simulink model "MECH6325_HW4_pblm3d"  (R2020a)
settings: Solver=VariableStepAuto  StartTime=0.0  StopTime=10.0  RelTol=1e-3
libraries: simulink x2, cstblocks x1
settings Model: Creator=Jonas  LastModifiedBy=Jonas

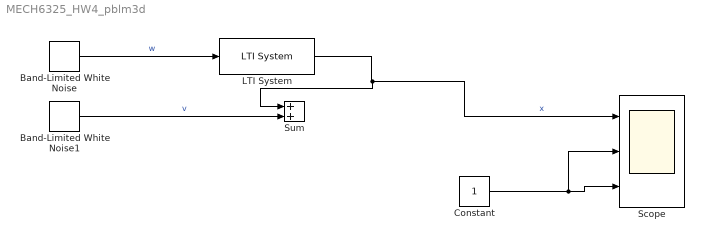
== system MECH6325_HW4_pblm3d ==
  Band-Limited White Noise : simulink/Sources/Band-Limited White Noise  Cov=[1]  Ts=0.1  seed=[23341]
  Band-Limited White Noise1 : simulink/Sources/Band-Limited White Noise  Cov=[1]  Ts=0.1  seed=[23341]
  Constant : Constant
  LTI System : cstblocks/LTI System  sys=sys  IC=[]
  Scope : Scope  NumInputPorts=3
  Sum : Sum
  wires:
  Band-Limited White Noise/1 -> LTI System/1  "w"
  LTI System/1 -> Sum/1, Scope/1  "x"
  Constant/1 -> Scope/3, Scope/2
  Band-Limited White Noise1/1 -> Sum/2  "v"
